simulink model "SpringPendulum"  (R2020b)
settings: Solver=VariableStepAuto  StartTime=0.0  StopTime=50  RelTol=1e-3
settings Model: Creator=Bk_space  LastModifiedBy=Bk_space

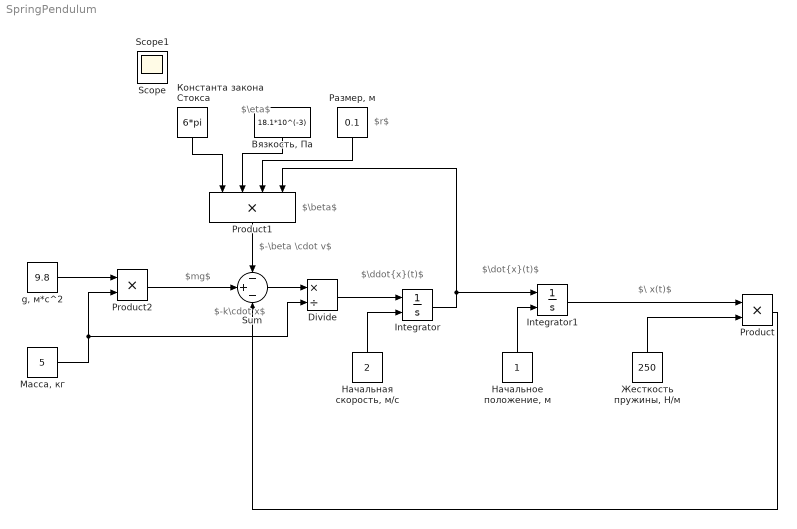
== system SpringPendulum ==
  note: $-k\cdot x$
  note: $mg$
  note: $r$
  note: $\eta$
  note: $-\beta \cdot v$
  note: $\beta$
  note: $\ddot{x}(t)$
  note: $\dot{x}(t)$
  note: $\ x(t)$
  Divide : Product  Inputs=*/
  Integrator : Integrator  InitialConditionSource=external  InitialCondition=-0.245
  Integrator1 : Integrator  InitialConditionSource=external
  Product : Product
  Product1 : Product  Inputs=4
  Product2 : Product
  Sum : Sum  Inputs=-+-
  "g, м*с^2" : Constant  Value=9.8
  "Вязкость, Па" : Constant  Value=18.1*10^(-3)
  "Жесткость пружины, Н/м" : Constant  Value=250
  Константа закона Стокса : Constant  Value=6*pi
  "Масса, кг" : Constant  Value=5
  "Начальная скорость, м/с" : Constant  Value=2
  "Начальное положение, м" : Constant
  "Размер, м" : Constant  Value=0.1
  Scope : Scope
  Scope1 : Scope
  wires:
  Integrator/1 -> Product1/4, Integrator1/1
  Product/1 -> Sum/3
  Integrator1/1 -> Product/1
  Sum/1 -> Divide/1
  Product1/1 -> Sum/1
  Divide/1 -> Integrator/1
  "Масса, кг"/1 -> Product2/2, Divide/2
  "Жесткость пружины, Н/м"/1 -> Product/2
  Константа закона Стокса/1 -> Product1/1
  "Вязкость, Па"/1 -> Product1/2
  "Размер, м"/1 -> Product1/3
  Product2/1 -> Sum/2
  "g, м*с^2"/1 -> Product2/1
  "Начальная скорость, м/с"/1 -> Integrator/2
  "Начальное положение, м"/1 -> Integrator1/2
